simulink model "empirical_fric"  (R2017a)
settings: Solver=FixedStepAuto  StartTime=0.0  StopTime=20  FixedStep=1e-3  RelTol=1e-3
libraries: simulink x2
settings Model: Creator=igricart  LastModifiedBy=igricart

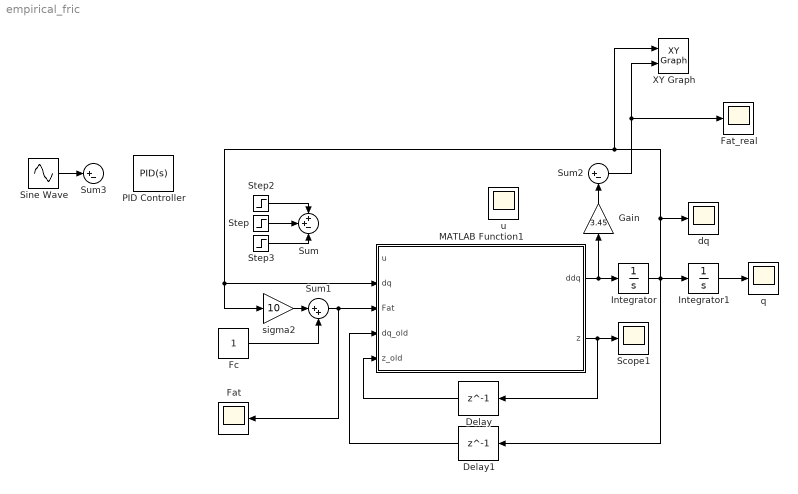
== system empirical_fric ==
  Delay : Delay  DelayLength=1
  Delay1 : Delay  DelayLength=1  InitialCondition=-1
  Fat : Scope
  Fat_real : Scope
  Fc : Constant
  Gain : Gain  Gain=3.45
  Integrator : Integrator
  Integrator1 : Integrator
  MATLAB Function1 : MATLAB Function  TreatAsAtomicUnit=on
  PID Controller : simulink/Continuous/PID Controller  Controller=PID  TimeDomain=Continuous-time  SampleTime=-1  IntegratorMethod=Forward Euler  FilterMethod=Forward Euler  Form=Parallel  UseFilter=on  ControllerParametersSource=internal  P=75  I=100  D=20  N=100  InitialConditionSource=internal  InitialConditionForIntegrator=0  InitialConditionForFilter=0  ExternalReset=none  LimitOutput=off  UpperSaturationLimit=inf  LowerSaturationLimit=-inf  LinearizeAsGain=on  AntiWindupMode=none  Kb=1  TrackingMode=off  Kt=1  PParamMin=[]  PParamMax=[]  IParamMin=[]  IParamMax=[]  DParamMin=[]  DParamMax=[]  NParamMin=[]  NParamMax=[]  KbParamMin=[]  KbParamMax=[]  KtParamMin=[]  KtParamMax=[]  POutMin=[]  POutMax=[]  IOutMin=[]  IOutMax=[]  DOutMin=[]  DOutMax=[]  NOutMin=[]  NOutMax=[]  KbOutMin=[]  KbOutMax=[]  KtOutMin=[]  KtOutMax=[]  IntegratorOutMin=[]  IntegratorOutMax=[]  FilterOutMin=[]  FilterOutMax=[]  SumOutMin=[]  SumOutMax=[]  SumI1OutMin=[]  SumI1OutMax=[]  SumI2OutMin=[]  SumI2OutMax=[]  SumI3OutMin=[]  SumI3OutMax=[]  SumDOutMin=[]  SumDOutMax=[]  SaturationOutMin=[]  SaturationOutMax=[]  IntegratorContinuousStateAttributes=''  IntegratorStateMustResolveToSignalObject=off  IntegratorRTWStateStorageClass=Auto  FilterContinuousStateAttributes=''  FilterStateMustResolveToSignalObject=off  FilterRTWStateStorageClass=Auto  DifferentiatorICPrevScaledInput=0  DifferentiatorOutMin=[]  DifferentiatorOutMax=[]  InitialConditionSetting=State (most efficient)
  Scope1 : Scope
  Sine Wave : Sin  Amplitude=5  Phase=pi/2  SampleTime=0
  Step : Step  SampleTime=0
  Step2 : Step  Time=6  After=10  SampleTime=0
  Step3 : Step  Time=7  After=9  SampleTime=0
  Sum : Sum  Inputs=++-
  Sum1 : Sum  Inputs=|++
  Sum2 : Sum  Inputs=|+-
  Sum3 : Sum  Inputs=|+-
  XY Graph : simulink/Sinks/XY Graph  xmin=-5  xmax=5  ymin=-5  ymax=7  st=-1
  dq : Scope
  q : Scope
  sigma2 : Gain  Gain=10
  u : Scope
  wires:
  MATLAB Function1/2(z) -> Scope1/1, Delay/1
  Delay/1 -> MATLAB Function1/5(z_old)
  Integrator/1 -> Integrator1/1, XY Graph/1, sigma2/1, MATLAB Function1/2(dq), dq/1, Delay1/1
  Sum1/1 -> MATLAB Function1/3(Fat), Fat/1
  Delay1/1 -> MATLAB Function1/4(dq_old)
  Step2/1 -> Sum/1
  Step/1 -> Sum/2
  Step3/1 -> Sum/3
  Fc/1 -> Sum1/2
  sigma2/1 -> Sum1/1
  ? -> MATLAB Function1/1(u), Sum2/1, u/1
  Integrator1/1 -> q/1
  MATLAB Function1/1(ddq) -> Integrator/1, Gain/1
  Sum2/1 -> Fat_real/1, XY Graph/2
  Gain/1 -> Sum2/2
  Sine Wave/1 -> Sum3/1

== matlab function empirical_fric/MATLAB Function1 ==
  data: u input; ddq output; dq input; Fat input; dq_old input; z_old input; z output
function [ddq, z] = friction( u, dq, Fat, dq_old, z_old)
    % z = static friction state, 1 = pre-slide regime
    
    Fs = 3;
    m = 3.45;
    M = 100*m;
    z = 0;
    
    % if system in slide regime, evaluate if velocity changed direction
    if z_old == 0
        %if so, pre-slide regime
        z = double(sign(dq) ~= sign(dq_old));
    elseif z_old == 1
        z = double(abs(u) <= Fs);
    end
    
    % to simulate stick-slip, the inertia changes according to regime
    ddq = u - Fat;
    if z == 0
        ddq = ddq/m;
    elseif z == 1
        ddq = ddq/M;
    end
